simulink library "lib_saturateMacroRobotPosition"  (R2023b)
settings: Solver=VariableStepAuto  StartTime=0.0  StopTime=10.0  RelTol=1e-3
undefined symbols (not defined in the file or in its folder): robotLowerLimits, robotLowerLimitsSlowDown, robotUpperLimits, robotUpperLimitsSlowDown
settings Model: Creator=muralikarnam  LastModifiedBy=User
settings SolverCC: AlgebraicLoopSolver=TrustRegion
settings DataIOCC: ReturnWorkspaceOutputs=off
settings DebuggingCC: UnconnectedInputMsg=warning  UnconnectedOutputMsg=warning  UnconnectedLineMsg=warning  ArithmeticOperatorsInVariantConditions=warning
settings ModelReferenceCC: EnableRefExpFcnMdlSchedulingChecks=on
settings SFSimCC: SimUseLocalCustomCode=off  CustomCodeUndefinedFunction=UseInterfaceOnly
settings RTWCC: RTWUseLocalCustomCode=off

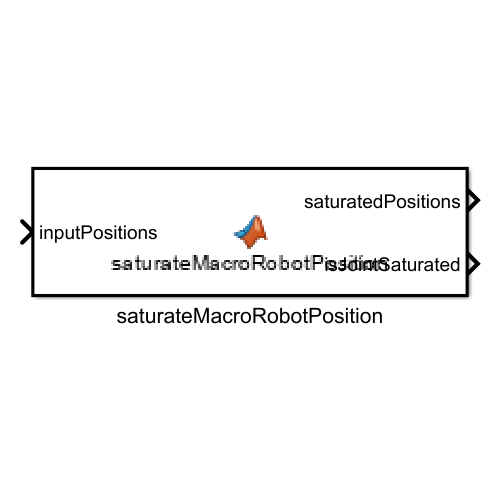
[thumbnail: Simulink's stored preview of the top-level diagram]
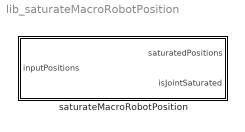
== system lib_saturateMacroRobotPosition ==
  saturateMacroRobotPosition : MATLAB Function  TreatAsAtomicUnit=on

== matlab function lib_saturateMacroRobotPosition/saturateMacroRobotPosition ==
  data: inputPositions input double size=[nJointsKuka 1]; saturatedPositions output double size=[nJointsKuka 1]; robotLowerLimits parameter double size=[nJointsKuka 1]; robotUpperLimits parameter double size=[nJointsKuka 1]; isJointSaturated output double size=[nJointsKuka 1]; robotLowerLimitsSlowDown parameter double size=[nJointsKuka 1]; robotUpperLimitsSlowDown parameter double size=[nJointsKuka 1]
function [saturatedPositions, isJointSaturated] = saturateMacroRobotPosition(inputPositions, robotLowerLimits, robotUpperLimits, robotLowerLimitsSlowDown, robotUpperLimitsSlowDown)

    [saturatedPositions, isJointSaturated]  = fun_SaturateMacroRobotPosition(inputPositions, robotUpperLimits, robotLowerLimits, robotLowerLimitsSlowDown, robotUpperLimitsSlowDown);
    
end
